simulink model "spring_mass_damper_simu"  (R2025b)
settings: Solver=VariableStepAuto  StartTime=0.0  StopTime=10.0  RelTol=1e-3
values from neighbouring files (symbols this model uses):
  A = [ ... (first row only)    [Lab_1.m]
  B = [0; 0; 0; 1/J1; 0; 0]    [Lab_1.m]
  C = [0 0 1 0 0 0]    [Lab_1.m]
  F = [ ... (first row only)    [Lab_1.m]
settings Model: Creator=DemoBox  LastModifiedBy=DemoBox

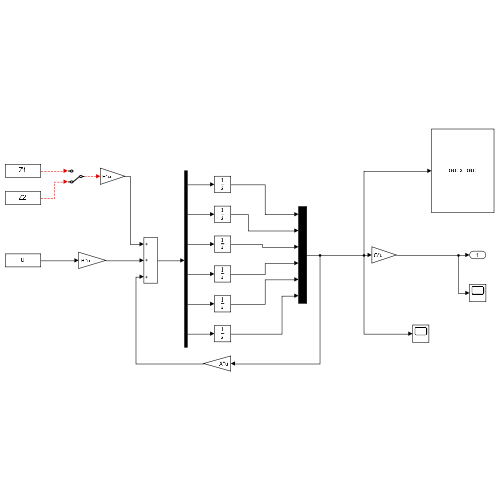
[thumbnail: Simulink's stored preview of the top-level diagram]
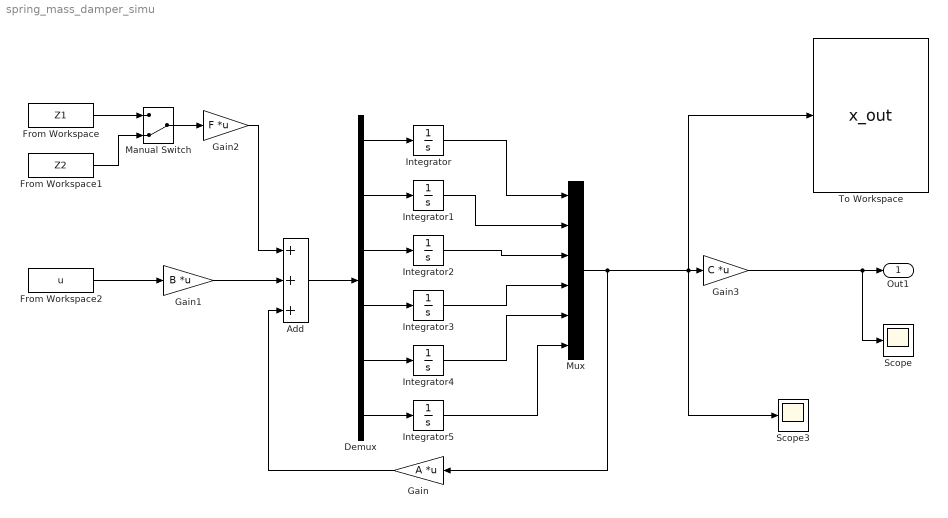
== system spring_mass_damper_simu ==
  Add : Sum  Inputs=+++
  Demux : Demux  Outputs=6
  From Workspace : FromWorkspace  VariableName=Z1
  From Workspace1 : FromWorkspace  VariableName=Z2
  From Workspace2 : FromWorkspace  VariableName=u
  Gain : Gain  Gain=A  Multiplication=Matrix(K*u)
  Gain1 : Gain  Gain=B  Multiplication=Matrix(K*u)
  Gain2 : Gain  Gain=F  Multiplication=Matrix(K*u)
  Gain3 : Gain  Gain=C  Multiplication=Matrix(K*u)
  Integrator{,1..5} (6 alike) : Integrator
  Manual Switch : ManualSwitch  CurrentSetting=0
  Mux : Mux  Inputs=6
  Scope : Scope
      settings: ActiveDisplayYMinimum=2.83958216055224  ActiveDisplayYMaximum=24.052024926023879
  Scope3 : Scope
      settings: ActiveDisplayYMinimum=18.639849141254739  ActiveDisplayYMaximum=23.222325515169974  DataLoggingVariableName=ScopeData3
  To Workspace : ToWorkspace  VariableName=x_out  SaveFormat=Structure With Time  SampleTime=-1
  Out1 : Outport
  wires:
  Integrator/1 -> Mux/1
  Integrator1/1 -> Mux/2
  Integrator2/1 -> Mux/3
  Integrator3/1 -> Mux/4
  Integrator4/1 -> Mux/5
  Integrator5/1 -> Mux/6
  Mux/1 -> To Workspace/1, Gain3/1, Scope3/1, Gain/1
  From Workspace2/1 -> Gain1/1
  Gain2/1 -> Add/1
  Gain1/1 -> Add/2
  Gain/1 -> Add/3
  Add/1 -> Demux/1
  Demux/1 -> Integrator/1
  Demux/2 -> Integrator1/1
  Demux/3 -> Integrator2/1
  Demux/4 -> Integrator3/1
  Demux/5 -> Integrator4/1
  Demux/6 -> Integrator5/1
  Gain3/1 -> Scope/1, Out1/1
  Manual Switch/1 -> Gain2/1
  From Workspace1/1 -> Manual Switch/2
  From Workspace/1 -> Manual Switch/1
